simulink model "Scenario_13_CoDeSys"  (R2012b)
settings: Solver=ode3  StartTime=0.0  StopTime=inf  FixedStep=Sample_Time_Model  RelTol=1e-3
PreLoadFcn:
  | Variablen_Scenario13
InitFcn:
  | BT = randperm(9);
values from neighbouring files (symbols this model uses):
  Band_Geschwindigkeit = 1.47    [Variablen_Scenario13.m]
  Band_Sensor_Hell_2_Z = -6.5    [Variablen_Scenario13.m]
  Band_Sensor_Hell_3_Z = -10.36    [Variablen_Scenario13.m]
  Band_Sensor_Hell_4_Z = -14.64    [Variablen_Scenario13.m]
  Band_Sensor_Tolerance_Z = 0.2    [Variablen_Scenario13.m]
  Bauteil_Fallgeschwindigkeit = 0.4    [Variablen_Scenario13.m]
  Bauteil_Farbe_Metall = [0.8 0.8 0.8]    [Variablen_Scenario13.m]
  Bauteil_Farbe_Schwarz = [0.2 0.2 0.2]    [Variablen_Scenario13.m]
  Bauteil_Farbe_Weiss = [1 1 0.2]    [Variablen_Scenario13.m]
  Kran_Dauer_90_Grad = 5    [Variablen_Scenario13.m]
  Kran_Drehwinkel_90_Grad = 8050    [Variablen_Scenario13.m]
  Kran_Sensor_Position_Delta = 0.07    [Variablen_Scenario13.m]
  Sample_Time_Model = 0.05    [Variablen_Scenario13.m]
  Sample_Time_Simulation = 0.1    [Variablen_Scenario13.m]
  Sensor_Band_Metall_1 = -6.5    [Variablen_Scenario13.m]
  Sensor_Band_Metall_2 = -10.36    [Variablen_Scenario13.m]
libraries: simulink x557, vrlib x13, opclib x7, rtwinlib x1
(part 3 of 10)

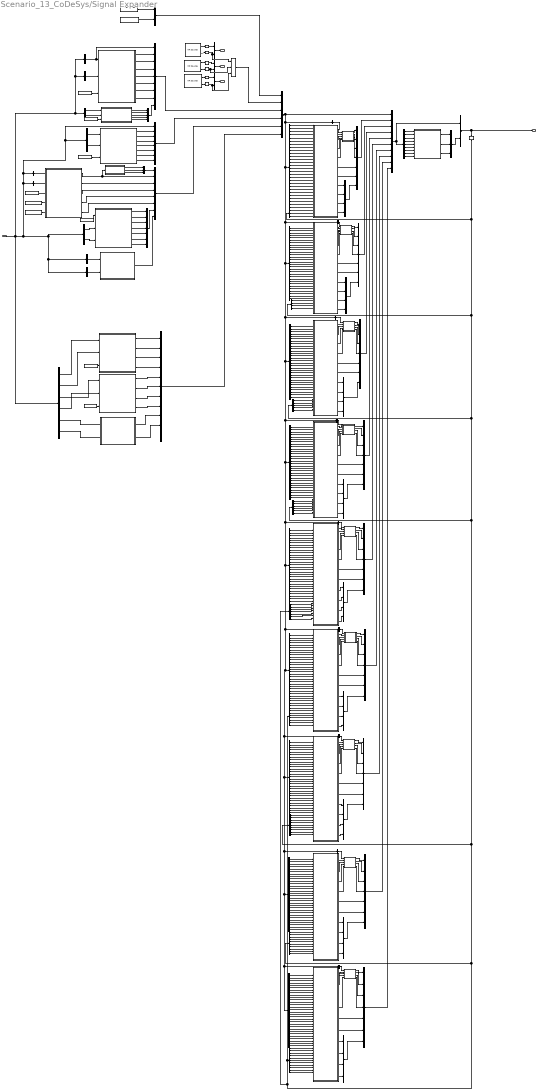
== system Scenario_13_CoDeSys/Signal Expander ==
  In : Inport
  BT_Lager_Status : Subsystem
  Band_Source : vrlib/VR Source  InstantiateOnLoad=on  SampleTime=Sample_Time_Simulation  ViewEnable=on  RemoteChange=off  RemoteView=off  FieldsRead=Switch_5.Button_State.1.1.1.logical#Switch_6.Switch_State.1.1.1.logical  WorldFileName=Visu_Sz_13.wrl  AutoView=off  VideoDimensions=[]  AllowVariableSize=off
  Band_Vor_Zurueck : Stateflow chart  TreatAsAtomicUnit=on
  Band_Zyl_1 : Stateflow chart  TreatAsAtomicUnit=on
  Band_Zyl_2 : Stateflow chart  TreatAsAtomicUnit=on
  Bauteil_1 : Stateflow chart  TreatAsAtomicUnit=on
  Bauteil_2 : Stateflow chart  TreatAsAtomicUnit=on
  Bauteil_3 : Stateflow chart  TreatAsAtomicUnit=on
  Bauteil_4 : Stateflow chart  TreatAsAtomicUnit=on
  Bauteil_5 : Stateflow chart  TreatAsAtomicUnit=on
  Bauteil_6 : Stateflow chart  TreatAsAtomicUnit=on
  Bauteil_7 : Stateflow chart  TreatAsAtomicUnit=on
  Bauteil_8 : Stateflow chart  TreatAsAtomicUnit=on
  Bauteil_9 : Stateflow chart  TreatAsAtomicUnit=on
  Bauteil_Fallgeschwindigkeit : Constant  Value=Bauteil_Fallgeschwindigkeit
  Berechne Band Geschwindigkeit : Subsystem
  Bus Creator : BusCreator  Inputs=5
  Bus Creator1 : BusCreator  Inputs=9
  Bus Creator10 : BusCreator  Inputs=10
  Bus Creator{9,11,21,24,26,29,31,33,35} (9 alike) : BusCreator
  Bus Creator{7..8,12,22,25,27..28,30,32,34} (10 alike) : BusCreator  Inputs=7
  Bus Creator13 : BusCreator  Inputs=3
  Bus Creator{14,18..19,23,36} (5 alike) : BusCreator  Inputs=2
  Bus Creator2 : BusCreator  Inputs=6
  Bus Creator3 : BusCreator  Inputs=8
  Bus Creator4 : BusCreator  Inputs=8
  Bus Creator5 : BusCreator  Inputs=11
  Bus Creator6 : BusCreator  Inputs=3
  Bus Selector1 : BusSelector  OutputSignals=Lager.Lager_X_Achse,Lager.Lager_Ver_Ausgefahren,Kran.Kran_Sensoren.Sensor_Kran_Stellung_Lager,Kran.Kran_Sensoren.Sensor_Kran_Stellung_Band,Kran.Kran_Sensoren.Sensor_Kran_Stellung_Stempel,Kran.Kran_Zyl.Kran_Zyl_Oben,Kran.Kran_Zyl.Kran_Zyl_Unten,Kran.Kran_Sauger,Kran.Kran_Zyl.Kran_Hochheben,Kran.Kran_Zyl.Kran_Runterlassen,Kran.Kran_Drehen_Links_FS,Kran.Kran_Drehen_Rechts_FS,Stempel.Stempel_Halterung_Ausfahren_FS,Stempel.Stempel_Halterung_Einfahren_FS,Band.Band_Vor_FS,Band.Band_Zurueck_FS,Band.Band_Zyl_1_X_Achse,Band.Band_Zyl_2_X_Achse,Lager.Lager_Ver_Ausfahren,Lager.Lager_Vereinzler_Schritt_Aus,Kran.Kran_Zyl.Kran_Zyl_Schritt_Hoch,Kran.Kran_Zyl.Kran_Zyl_Schritt_Runter,Kran.Kran_Drehen_Schritt,Stempel.Stempel_Halterung_Schritt_Aus,Stempel.Stempel_Halterung_Schritt_Ein,Band.Band_Zyl_1_Schritt,Band.Band_Zyl_2_Schritt,Konstante.Band_Geschwindigkeit
  Bus Selector10 : BusSelector  OutputSignals=Stempel.Stempel_Halterung_ausfahren
  Bus Selector11 : BusSelector  OutputSignals=Stempel.Stempel_Halterung_einfahren
  Bus Selector12 : BusSelector  OutputSignals=Stempel.Stempel_einfahren,Stempel.Stempel_ausfahren
  Bus Selector13 : BusSelector  OutputSignals=Kran.Kran_Sauger_An
  Bus Selector14 : BusSelector  OutputSignals=Kran.Kran_Sauger_Aus
  Bus Selector15 : BusSelector  OutputSignals=Kran.Kran_einfahren,Kran.Kran_ausfahren
  Bus Selector16 : BusSelector  OutputSignals=Kran.Kran_Drehen_Links
  Bus Selector17 : BusSelector  OutputSignals=Kran.Kran_Drehen_Rechts
  Bus Selector18 : BusSelector  OutputSignals=Lager.Lager_Zyl_einfahren,Lager.Lager_Zyl_ausfahren
  Bus Selector19 : BusSelector  OutputSignals=Lager.Lager_1_Status,Lager.Lager_2_Status,Lager.Lager_3_Status,Stempelanlage_BT.Bauteil_1.BT_1_Bereit,Stempelanlage_BT.Bauteil_2.BT_2_Bereit
  Bus Selector{2,9,21,23,25,31..32,34} (8 alike) : BusSelector  OutputSignals=Lager.Lager_X_Achse,Lager.Lager_Ver_Eingefahren,Lager.Lager_Ver_Ausgefahren,Kran.Kran_Sensoren.Sensor_Kran_Stellung_Lager,Kran.Kran_Sensoren.Sensor_Kran_Stellung_Band,Kran.Kran_Sensoren.Sensor_Kran_Stellung_Stempel,Kran.Kran_Zyl.Kran_Zyl_Oben,Kran.Kran_Zyl.Kran_Zyl_Unten,Kran.Kran_Sauger,Kran.Kran_Zyl.Kran_Hochheben,Kran.Kran_Zyl.Kran_Runterlassen,Kran.Kran_Drehen_Links_FS,Kran.Kran_Drehen_Rechts_FS,Stempel.Stempel_Halterung_Ausfahren_FS,Stempel.Stempel_Halterung_Einfahren_FS,Band.Band_Vor_FS,Band.Band_Zurueck_FS,Band.Band_Zyl_1_X_Achse,Band.Band_Zyl_2_X_Achse,Lager.Lager_Ver_Ausfahren,Lager.Lager_Vereinzler_Schritt_Aus,Kran.Kran_Zyl.Kran_Zyl_Schritt_Hoch,Kran.Kran_Zyl.Kran_Zyl_Schritt_Runter,Kran.Kran_Drehen_Schritt,Stempel.Stempel_Halterung_Schritt_Aus,Stempel.Stempel_Halterung_Schritt_Ein,Band.Band_Zyl_1_Schritt,Band.Band_Zyl_2_Schritt,Konstante.Band_Geschwindigkeit,Konstante.Bauteil_Fallgeschwindigkeit
  Bus Selector20 : BusSelector  OutputSignals=Lager.Lager_1_Status,Lager.Lager_2_Status,Lager.Lager_3_Status,Stempelanlage_BT.Bauteil_1.BT_1_Bereit,Stempelanlage_BT.Bauteil_2.BT_2_Bereit,Stempelanlage_BT.Bauteil_3.BT_3_Bereit
  Bus Selector22 : BusSelector  OutputSignals=Lager.Lager_1_Status,Lager.Lager_2_Status,Lager.Lager_3_Status,Stempelanlage_BT.Bauteil_1.BT_1_Bereit,Stempelanlage_BT.Bauteil_2.BT_2_Bereit,Stempelanlage_BT.Bauteil_3.BT_3_Bereit,Stempelanlage_BT.Bauteil_4.BT_4_Bereit
  Bus Selector24 : BusSelector  OutputSignals=Lager.Lager_1_Status,Lager.Lager_2_Status,Lager.Lager_3_Status,Stempelanlage_BT.Bauteil_1.BT_1_Bereit,Stempelanlage_BT.Bauteil_2.BT_2_Bereit,Stempelanlage_BT.Bauteil_3.BT_3_Bereit,Stempelanlage_BT.Bauteil_4.BT_4_Bereit,Stempelanlage_BT.Bauteil_5.BT_5_Bereit
  Bus Selector26 : BusSelector  OutputSignals=Band.Band_Zyl_1_einfahren,Band.Band_Zyl_1_ausfahren,Band.Band_Zyl_2_einfahren,Band.Band_Zyl_2_ausfahren,Band.Band_vor,Band.Band_zurueck
  Bus Selector{6,8,27..30,36..38} (9 alike) : BusSelector  OutputSignals=Notaus_Switch
  Bus Selector3 : BusSelector  OutputSignals=Lager.Lager_1_Status,Lager.Lager_2_Status,Lager.Lager_3_Status,Stempelanlage_BT.Bauteil_1.BT_1_Bereit
  Bus Selector33 : BusSelector  OutputSignals=Lager.Lager_1_Status,Lager.Lager_2_Status,Lager.Lager_3_Status,Stempelanlage_BT.Bauteil_1.BT_1_Bereit,Stempelanlage_BT.Bauteil_2.BT_2_Bereit,Stempelanlage_BT.Bauteil_3.BT_3_Bereit,Stempelanlage_BT.Bauteil_4.BT_4_Bereit,Stempelanlage_BT.Bauteil_5.BT_5_Bereit,Stempelanlage_BT.Bauteil_6.BT_6_Bereit,Stempelanlage_BT.Bauteil_7.BT_7_Bereit
  Bus Selector35 : BusSelector  OutputSignals=Lager.Lager_1_Status,Lager.Lager_2_Status,Lager.Lager_3_Status,Stempelanlage_BT.Bauteil_1.BT_1_Bereit,Stempelanlage_BT.Bauteil_2.BT_2_Bereit,Stempelanlage_BT.Bauteil_3.BT_3_Bereit,Stempelanlage_BT.Bauteil_4.BT_4_Bereit,Stempelanlage_BT.Bauteil_5.BT_5_Bereit,Stempelanlage_BT.Bauteil_6.BT_6_Bereit,Stempelanlage_BT.Bauteil_7.BT_7_Bereit,Stempelanlage_BT.Bauteil_8.BT_8_Bereit
  Bus Selector4 : BusSelector  OutputSignals=Bauteil_1.BT_1_Lager,Bauteil_2.BT_2_Lager,Bauteil_3.BT_3_Lager,Bauteil_4.BT_4_Lager,Bauteil_5.BT_5_Lager,Bauteil_6.BT_6_Lager,Bauteil_7.BT_7_Lager,Bauteil_8.BT_8_Lager,Bauteil_9.BT_9_Lager
  Bus Selector5 : BusSelector  OutputSignals=Lager.Lager_1_Status,Lager.Lager_2_Status,Lager.Lager_3_Status
  Bus Selector7 : BusSelector  OutputSignals=Lager.Lager_1_Status,Lager.Lager_2_Status,Lager.Lager_3_Status,Stempelanlage_BT.Bauteil_1.BT_1_Bereit,Stempelanlage_BT.Bauteil_2.BT_2_Bereit,Stempelanlage_BT.Bauteil_3.BT_3_Bereit,Stempelanlage_BT.Bauteil_4.BT_4_Bereit,Stempelanlage_BT.Bauteil_5.BT_5_Bereit,Stempelanlage_BT.Bauteil_6.BT_6_Bereit
  Constant{14..17,24..25,30} (7 alike) : Constant  Value=Sample_Time_Model
  Constant31 : Constant  Value=Kran_Drehwinkel_90_Grad
  Constant32 : Constant  Value=Kran_Dauer_90_Grad
  Halterung_Stempel : Stateflow chart  TreatAsAtomicUnit=on
  Kran : Stateflow chart  TreatAsAtomicUnit=on
  Kran_Position_Sensor : Subsystem
  Kran_Sauger : Stateflow chart  TreatAsAtomicUnit=on
  Kran_Zylinder : Stateflow chart  TreatAsAtomicUnit=on
  Lager : Stateflow chart  TreatAsAtomicUnit=on
  Lager_Source : vrlib/VR Source  InstantiateOnLoad=on  SampleTime=Sample_Time_Simulation  ViewEnable=on  RemoteChange=off  RemoteView=off  FieldsRead=Switch_1.Button_State.1.1.1.logical#Switch_2.Switch_State.1.1.1.logical  WorldFileName=Visu_Sz_13.wrl  AutoView=off  VideoDimensions=[]  AllowVariableSize=off
  Logical Operator : Logic  Operator=OR  Inputs=3  AllPortsSameDT=off  OutDataTypeStr=boolean
  Memory4 : Memory
  Rate Transition{1..6} (6 alike) : RateTransition
  Stempel_Source : vrlib/VR Source  InstantiateOnLoad=on  SampleTime=Sample_Time_Simulation  ViewEnable=on  RemoteChange=off  RemoteView=off  FieldsRead=Switch_3.Button_State.1.1.1.logical#Switch_4.Switch_State.1.1.1.logical  WorldFileName=Visu_Sz_13.wrl  AutoView=off  VideoDimensions=[]  AllowVariableSize=off
  Subsystem : Subsystem
  Subsystem1 : Subsystem
  Subsystem2 : Subsystem
  Subsystem3 : Subsystem
  Subsystem4 : Subsystem
  Subsystem5 : Subsystem
  Subsystem6 : Subsystem
  Subsystem7 : Subsystem
  Subsystem8 : Subsystem
  Zylinder_Stempel : Stateflow chart  TreatAsAtomicUnit=on
  Band_Schalter : Outport
  Lager_Schalter : Outport  Port=2
  Stempel_Schalter : Outport  Port=3
  Bauteil_Ausgang : Outport  Port=4
  wires:
  Halterung_Stempel/1(Halterung_X_Achse) -> Bus Creator1/2  "Stempel_Halterung_X_Achse"
  Bus Creator1/1 -> Bus Creator2/3  "Stempel"
  Lager/1(Vereinzler_X_Achse) -> Bus Creator3/2  "Lager_X_Achse"
  Bus Creator3/1 -> Bus Creator2/4  "Lager"
  Bus Selector18/2 -> Lager/2(Vereinzler_Ausfahren)  "<Lager_Zyl_ausfahren>"
  Bus Selector16/1 -> Kran/1(Kran_Drehen_Links)  "<Kran_Drehen_Links>"
  Bus Creator4/1 -> Bus Creator2/5  "Kran"
  Kran/1(Kran_Stellung) -> Kran_Position_Sensor/1(In), Bus Creator4/2  "Kran_Stellung"
  Bus Selector17/1 -> Kran/2(Kran_Drehen_Rechts)  "<Kran_Drehen_Rechts>"
  Bus Creator5/1 -> Bus Creator2/6  "Band"
  Zylinder_Stempel/1(Zylinder_Y_Achse) -> Bus Creator/1  "Stempel_Zyl_Y"
  Band_Zyl_1/1(Zyl_1_X_Achse) -> Bus Creator5/1  "Band_Zyl_1_X_Achse"
  Band_Zyl_2/2(Zyl_2_X_Achse) -> Bus Creator5/6  "Band_Zyl_2_X_Achse"
  Bus Selector15/1 -> Kran_Zylinder/2(Kran_Zyl_Runter)  "<Kran_einfahren>"
  Kran_Sauger/1(Kran_Sauger_On) -> Bus Creator4/8  "Kran_Sauger"
  Bus Selector13/1 -> Kran_Sauger/1(Kran_Sauger_An)  "<Kran_Sauger_An>"
  Bus Selector14/1 -> Kran_Sauger/2(Kran_Sauger_Aus)  "<Kran_Sauger_Aus>"
  Kran_Position_Sensor/2(Sensor_Kran_Stellung_Band) -> Bus Creator6/2  "Sensor_Kran_Stellung_Band"
  Kran_Position_Sensor/1(Sensor_Kran_Stellung_Lager) -> Bus Creator6/1  "Sensor_Kran_Stellung_Lager"
  Kran_Position_Sensor/3(Sensor_Kran_Stellung_Stempel) -> Bus Creator6/3  "Sensor_Kran_Stellung_Stempel"
  Bus Creator6/1 -> Bus Creator4/1  "Kran_Sensoren"
  Kran_Zylinder/1(Kran_Zyl_Y_Achse) -> Bus Creator7/1  "Kran_Zyl_Y_Achse"
  Kran_Zylinder/2(Kran_Zyl_Oben) -> Bus Creator7/2  "Kran_Zyl_Oben"
  Kran_Zylinder/3(Kran_Zyl_Unten) -> Bus Creator7/3  "Kran_Zyl_Unten"
  Bus Creator7/1 -> Bus Creator4/7  "Kran_Zyl"
  Bus Selector10/1 -> Bus Creator1/1, Halterung_Stempel/1(Halterung_Ausfahren)  "<Stempel_Halterung_ausfahren>"
  Bus Selector11/1 -> Halterung_Stempel/2(Halterung_Einfahren)  "<Stempel_Halterung_einfahren>"
  Bus Selector12/1 -> Zylinder_Stempel/1(Stempel_Einfahren)  "<Stempel_einfahren>"
  Halterung_Stempel/2(Stempel_Halterung_Ausgefahren) -> Bus Creator1/3  "Stempel_Halterung_Ausgefahren"
  Halterung_Stempel/3(Stempel_Halterung_Eingefahren) -> Bus Creator1/4  "Stempel_Halterung_Eingefahren"
  Zylinder_Stempel/2(Stempel_Zylinder_Eingefahren) -> Bus Creator/2  "Stempel_Zyl_Eingefahren"
  Zylinder_Stempel/3(Stempel_Zylinder_Ausgefahren) -> Bus Creator/3  "Stempel_Zyl_Ausgefahren"
  Bus Creator/1 -> Bus Creator1/9  "Stempel_Zyl"
  Bauteil_1/1(BT_Y_Achse) -> Subsystem/2(BT_Y_In)  "BT_1_Y_Achse"
  Bauteil_1/5(BT_X_Achse) -> Bus Creator8/5  "BT_1_X_Achse"
  Bauteil_1/6(BT_Z_Achse) -> Bus Creator8/6  "BT_1_Z_Achse"
  Bus Selector1/1 -> Bauteil_1/1(Lager_X_Achse)  "<Lager_X_Achse>"
  Lager/2(Vereinzler_Eingefahren) -> Bus Creator3/3  "Lager_Ver_Eingefahren"
  Lager/3(Vereinzler_Ausgefahren) -> Bus Creator3/4  "Lager_Ver_Ausgefahren"
  Bus Selector1/2 -> Bauteil_1/2(Lager_Ver_Ausgefahren)  "<Lager_Ver_Ausgefahren>"
  Bus Selector1/3 -> Bauteil_1/3(Kran_Stellung_Lager)  "<Sensor_Kran_Stellung_Lager>"
  Bus Selector1/4 -> Bauteil_1/4(Kran_Stellung_Band)  "<Sensor_Kran_Stellung_Band>"
  Bus Selector1/5 -> Bauteil_1/5(Kran_Stellung_Stempel)  "<Sensor_Kran_Stellung_Stempel>"
  Bus Selector1/6 -> Bauteil_1/6(Kran_Zyl_Oben)  "<Kran_Zyl_Oben>"
  Bus Selector1/7 -> Bauteil_1/7(Kran_Zyl_Unten)  "<Kran_Zyl_Unten>"
  Kran_Zylinder/4(Kran_Hochheben) -> Bus Creator7/4  "Kran_Hochheben"
  Kran_Zylinder/5(Kran_Runterlassen) -> Bus Creator7/5  "Kran_Runterlassen"
  Bus Selector1/9 -> Bauteil_1/9(Kran_Hochheben)  "<Kran_Hochheben>"
  Bus Selector1/10 -> Bauteil_1/10(Kran_Runterlassen)  "<Kran_Runterlassen>"
  Kran/2(Kran_Drehen_Links_FS) -> Bus Creator4/3  "Kran_Drehen_Links_FS"
  Kran/3(Kran_Drehen_Rechts_FS) -> Bus Creator4/4  "Kran_Drehen_Rechts_FS"
  Bus Selector1/11 -> Bauteil_1/11(Kran_Drehen_Links)  "<Kran_Drehen_Links_FS>"
  Bus Selector1/12 -> Bauteil_1/12(Kran_Drehen_Rechts)  "<Kran_Drehen_Rechts_FS>"
  Halterung_Stempel/4(Stempel_Halterung_Ausfahren_FS) -> Bus Creator1/5  "Stempel_Halterung_Ausfahren_FS"
  Halterung_Stempel/5(Stempel_Halterung_Einfahren_FS) -> Bus Creator1/6  "Stempel_Halterung_Einfahren_FS"
  Bus Selector1/13 -> Bauteil_1/13(Stempel_Halterung_Ausfahren)  "<Stempel_Halterung_Ausfahren_FS>"
  Bus Selector1/14 -> Bauteil_1/14(Stempel_Halterung_Einfahren)  "<Stempel_Halterung_Einfahren_FS>"
  Band_Vor_Zurueck/1(Band_Vor_FS) -> Bus Creator5/9  "Band_Vor_FS"
  Band_Vor_Zurueck/2(Band_Zurueck_FS) -> Bus Creator5/10  "Band_Zurueck_FS"
  Bus Selector1/15 -> Bauteil_1/15(Band_Vor)  "<Band_Vor_FS>"
  Bus Selector1/16 -> Bauteil_1/16(Band_Zurueck)  "<Band_Zurueck_FS>"
  Bus Selector1/17 -> Bauteil_1/17(Band_Zyl_1_X_Achse)  "<Band_Zyl_1_X_Achse>"
  Bus Selector1/18 -> Bauteil_1/18(Band_Zyl_2_X_Achse)  "<Band_Zyl_2_X_Achse>"
  Bauteil_1/7(BT_Rotation_1) -> Bus Creator9/1
  Bauteil_1/8(BT_Rotation_2) -> Bus Creator9/2
  Bauteil_1/9(BT_Rotation_3) -> Bus Creator9/3
  Bauteil_1/10(BT_Rotation_4) -> Bus Creator9/4
  Bus Creator9/1 -> Bus Creator8/7  "BT_1_Rotation"
  Lager/5(Lager_Ver_Ausfahren) -> Bus Creator3/6  "Lager_Ver_Ausfahren"
  Lager/4(Lager_Ver_Einfahren) -> Bus Creator3/5  "Lager_Ver_Einfahren"
  Bus Selector1/19 -> Bauteil_1/19(Lager_Ver_Ausfahren)  "<Lager_Ver_Ausfahren>"
  Bus Creator8/1 -> Bus Creator10/2  "Bauteil_1"
  Bus Creator10/1 -> Bus Creator14/1, Bus Selector4/1  "Stempelanlage_BT"
  Bauteil_2/7(BT_Rotation_1) -> Bus Creator11/1
  Bauteil_2/8(BT_Rotation_2) -> Bus Creator11/2
  Bauteil_2/9(BT_Rotation_3) -> Bus Creator11/3
  Bauteil_2/10(BT_Rotation_4) -> Bus Creator11/4
  Bauteil_2/5(BT_X_Achse) -> Bus Creator12/5  "BT_2_X_Achse"
  Bauteil_2/1(BT_Y_Achse) -> Subsystem8/2(BT_Y_In)  "BT_2_Y_Achse"
  Bauteil_2/6(BT_Z_Achse) -> Bus Creator12/6  "BT_2_Z_Achse"
  Bus Creator11/1 -> Bus Creator12/7  "BT_2_Rotation"
  Bus Creator12/1 -> Bus Creator10/3  "Bauteil_2"
  Bauteil_1/4(BT_1_Bereit) -> Subsystem/5(BT_Bereit)
  Bauteil_1/2(BT_1_Lager) -> Subsystem/3(BT_Lager_In)  "BT_1_Lager"
  Bauteil_2/2(BT_Lager) -> Subsystem8/3(BT_Lager_In)
  Bus Selector4/1 -> BT_Lager_Status/1(BT_1_Lager_Position)  "<BT_1_Lager>"
  Bus Selector4/2 -> BT_Lager_Status/2(BT_2_Lager_Position)  "<BT_2_Lager>"
  BT_Lager_Status/1(Lager_1_Status) -> Bus Creator13/1  "Lager_1_Status"
  BT_Lager_Status/2(Lager_2_Status) -> Bus Creator13/2  "Lager_2_Status"
  BT_Lager_Status/3(Lager_3_Status) -> Bus Creator13/3  "Lager_3_Status"
  Bus Creator14/1 -> Bauteil_Ausgang/1, Memory4/1
  Bus Creator13/1 -> Bus Creator14/2  "Lager"
  Bauteil_2/4(BT_Bereit) -> Subsystem8/5(BT_Bereit)
  Bus Selector5/1 -> Bauteil_1/29(Lager_1_Status)  "<Lager_1_Status>"
  Bus Selector5/2 -> Bauteil_1/30(Lager_2_Status)  "<Lager_2_Status>"
  Bus Selector5/3 -> Bauteil_1/31(Lager_3_Status)  "<Lager_3_Status>"
  In/1 -> Bus Selector26/1, Bus Selector10/1, Bus Selector11/1, Bus Selector12/1, Bus Creator3/1, Bus Selector18/1, Bus Selector16/1, Bus Selector17/1, Bus Selector13/1, Bus Selector14/1, Bus Selector15/1  "Kran_Lager_FS"
  Band_Zyl_2/4(Band_Zyl_2_Ausgefahren) -> Bus Creator5/8  "Band_Zyl_2_Ausgefahren"
  Band_Zyl_2/3(Band_Zyl_2_Eingefahren) -> Bus Creator5/7  "Band_Zyl_2_Eingefahren"
  Band_Zyl_1/2(Band_Zyl_1_Eingefahren) -> Bus Creator5/2  "Band_Zyl_1_Eingefahren"
  Band_Zyl_1/3(Band_Zyl_1_Ausgefahren) -> Bus Creator5/3  "Band_Zyl_1_Ausgefahren"
  Bauteil_1/3(Kran_Sauger_BT) -> Subsystem/4(BT_angesaugt_in)  "Kran_Sauger_BT_1"
  Bauteil_2/3(Kran_Sauger_BT) -> Subsystem8/4(BT_angesaugt_in)
  Bus Creator21/1 -> Bus Creator22/7  "BT_3_Rotation"
  Bauteil_3/5(BT_X_Achse) -> Bus Creator22/5  "BT_3_X_Achse"
  Bauteil_3/1(BT_Y_Achse) -> Subsystem1/2(BT_Y_In)
  Bauteil_3/6(BT_Z_Achse) -> Bus Creator22/6  "BT_3_Z_Achse"
  Bauteil_3/4(BT_Bereit) -> Subsystem1/5(BT_Bereit)
  Bauteil_3/2(BT_Lager) -> Subsystem1/3(BT_Lager_In)
  Bauteil_3/3(Kran_Sauger_BT) -> Subsystem1/4(BT_angesaugt_in)
  Bauteil_3/7(BT_Rotation_1) -> Bus Creator21/1
  Bauteil_3/8(BT_Rotation_2) -> Bus Creator21/2
  Bauteil_3/9(BT_Rotation_3) -> Bus Creator21/3
  Bauteil_3/10(BT_Rotation_4) -> Bus Creator21/4
  Bus Creator22/1 -> Bus Creator10/4  "Bauteil_3"
  Bus Selector4/3 -> BT_Lager_Status/3(BT_3_Lager_Position)  "<BT_3_Lager>"
  Constant14/1 -> Lager/3(Sample_Time)
  Constant15/1 -> Halterung_Stempel/3(Sample_Time)
  Constant16/1 -> Zylinder_Stempel/3(Sample_Time)
  Constant17/1 -> Kran_Zylinder/1(Sample_Time)
  Constant24/1 -> Kran/3(Sample_Time)
  Constant25/1 -> Band_Zyl_1/3(Sample_Time)
  Constant30/1 -> Band_Zyl_2/3(Sample_Time)
  Halterung_Stempel/6(Schrittgroesse_Ausfahren) -> Bus Creator1/7  "Stempel_Halterung_Schritt_Aus"
  Halterung_Stempel/7(Schrittgroesse_Einfahren) -> Bus Creator1/8  "Stempel_Halterung_Schritt_Ein"
  Zylinder_Stempel/4(Schrittgroesse_Ausfahren) -> Bus Creator/4  "Stempel_Zyl_Schritt_Aus"
  Zylinder_Stempel/5(Schrittgroesse_Einfahren) -> Bus Creator/5  "Stempel_Zyl_Schritt_Ein"
  Lager/6(Schrittgroesse_Ausfahren) -> Bus Creator3/7  "Lager_Vereinzler_Schritt_Aus"
  Lager/7(Schrittgroesse_Einfahren) -> Bus Creator3/8  "Lager_Vereinzler_Schritt_Ein"
  Kran/4(Schrittgroesse_Drehen) -> Bus Creator4/5  "Kran_Drehen_Schritt"
  Kran_Zylinder/6(Schrittgroesse_Ausfahren) -> Bus Creator7/6  "Kran_Zyl_Schritt_Runter"
  Kran_Zylinder/7(Schrittgroesse_Einfahren) -> Bus Creator7/7  "Kran_Zyl_Schritt_Hoch"
  Band_Zyl_2/1(Schrittgroesse) -> Bus Creator5/5  "Band_Zyl_2_Schritt"
  Band_Zyl_1/4(Schrittgroesse) -> Bus Creator5/4  "Band_Zyl_1_Schritt"
  Bus Selector1/20 -> Bauteil_1/20(Lager_Vereinzler_Schritt_Aus)  "<Lager_Vereinzler_Schritt_Aus>"
  Bus Selector1/22 -> Bauteil_1/22(Kran_Zyl_Schritt_Runter)  "<Kran_Zyl_Schritt_Runter>"
  Bus Selector1/21 -> Bauteil_1/21(Kran_Zyl_Schritt_Hoch)  "<Kran_Zyl_Schritt_Hoch>"
  Bus Selector1/23 -> Bauteil_1/23(Kran_Drehen_Schritt)  "<Kran_Drehen_Schritt>"
  Bus Selector1/24 -> Bauteil_1/24(Stempel_Halterung_Schritt_Aus)  "<Stempel_Halterung_Schritt_Aus>"
  Bus Selector1/25 -> Bauteil_1/25(Stempel_Halterung_Schritt_Ein)  "<Stempel_Halterung_Schritt_Ein>"
  Bus Selector1/8 -> Bauteil_1/8(Kran_Sauger)  "<Kran_Sauger>"
  Bus Selector1/26 -> Bauteil_1/26(Band_Zyl_1_Schritt)  "<Band_Zyl_1_Schritt>"
  Bus Selector1/27 -> Bauteil_1/27(Band_Zyl_2_Schritt)  "<Band_Zyl_2_Schritt>"
  Berechne Band Geschwindigkeit/1(Band_Geschwindigkeit) -> Bus Creator23/1  "Band_Geschwindigkeit"
  Bauteil_Fallgeschwindigkeit/1 -> Bus Creator23/2  "Bauteil_Fallgeschwindigkeit"
  Bus Creator23/1 -> Bus Creator2/1  "Konstante"
  Bus Selector1/28 -> Bauteil_1/28(Band_Geschwindigkeit)  "<Band_Geschwindigkeit>"
  Bus Selector2/10 -> Bauteil_2/10(Kran_Hochheben)  "<Kran_Hochheben>"
  Bus Selector2/28 -> Bauteil_2/28(Band_Zyl_2_Schritt)  "<Band_Zyl_2_Schritt>"
  Bus Selector2/11 -> Bauteil_2/11(Kran_Runterlassen)  "<Kran_Runterlassen>"
  Bus Selector2/7 -> Bauteil_2/7(Kran_Zyl_Oben)  "<Kran_Zyl_Oben>"
  Bus Selector2/3 -> Bauteil_2/3(Lager_Ver_Ausgefahren)  "<Lager_Ver_Ausgefahren>"
  Bus Selector3/2 -> Bauteil_2/32(Lager_2_Status)  "<Lager_2_Status>"
  Bus Selector3/1 -> Bauteil_2/31(Lager_1_Status)  "<Lager_1_Status>"
  Bus Selector2/4 -> Bauteil_2/4(Kran_Stellung_Lager)  "<Sensor_Kran_Stellung_Lager>"
  Bus Selector2/30 -> Bauteil_2/30(Bauteil_Fallgeschwindigkeit)  "<Bauteil_Fallgeschwindigkeit>"
  Bus Selector2/21 -> Bauteil_2/21(Lager_Vereinzler_Schritt_Aus)  "<Lager_Vereinzler_Schritt_Aus>"
  Bus Selector2/8 -> Bauteil_2/8(Kran_Zyl_Unten)  "<Kran_Zyl_Unten>"
  Bus Selector2/23 -> Bauteil_2/23(Kran_Zyl_Schritt_Runter)  "<Kran_Zyl_Schritt_Runter>"
  Bus Selector2/6 -> Bauteil_2/6(Kran_Stellung_Stempel)  "<Sensor_Kran_Stellung_Stempel>"
  Bus Selector2/1 -> Bauteil_2/1(Lager_X_Achse)  "<Lager_X_Achse>"
  Bus Selector2/27 -> Bauteil_2/27(Band_Zyl_1_Schritt)  "<Band_Zyl_1_Schritt>"
  Bus Selector2/13 -> Bauteil_2/13(Kran_Drehen_Rechts)  "<Kran_Drehen_Rechts_FS>"
  Bus Selector2/15 -> Bauteil_2/15(Stempel_Halterung_Einfahren)  "<Stempel_Halterung_Einfahren_FS>"
  Bus Selector2/19 -> Bauteil_2/19(Band_Zyl_2_X_Achse)  "<Band_Zyl_2_X_Achse>"
  Bus Selector2/18 -> Bauteil_2/18(Band_Zyl_1_X_Achse)  "<Band_Zyl_1_X_Achse>"
  Bus Selector2/22 -> Bauteil_2/22(Kran_Zyl_Schritt_Hoch)  "<Kran_Zyl_Schritt_Hoch>"
  Bus Selector2/20 -> Bauteil_2/20(Lager_Ver_Ausfahren)  "<Lager_Ver_Ausfahren>"
  Bus Selector2/17 -> Bauteil_2/17(Band_Zurueck)  "<Band_Zurueck_FS>"
  Bus Selector2/24 -> Bauteil_2/24(Kran_Drehen_Schritt)  "<Kran_Drehen_Schritt>"
  Bus Selector2/14 -> Bauteil_2/14(Stempel_Halterung_Ausfahren)  "<Stempel_Halterung_Ausfahren_FS>"
  Bus Selector2/16 -> Bauteil_2/16(Band_Vor)  "<Band_Vor_FS>"
  Bus Selector2/25 -> Bauteil_2/25(Stempel_Halterung_Schritt_Aus)  "<Stempel_Halterung_Schritt_Aus>"
  Bus Selector2/2 -> Bauteil_2/2(Lager_Ver_Eingefahren)  "<Lager_Ver_Eingefahren>"
  Bus Selector2/26 -> Bauteil_2/26(Stempel_Halterung_Schritt_Ein)  "<Stempel_Halterung_Schritt_Ein>"
  Bus Selector2/9 -> Bauteil_2/9(Kran_Sauger)  "<Kran_Sauger>"
  Bus Selector2/29 -> Bauteil_2/29(Band_Geschwindigkeit)  "<Band_Geschwindigkeit>"
  Bus Selector3/3 -> Bauteil_2/33(Lager_3_Status)  "<Lager_3_Status>"
  Bus Selector2/12 -> Bauteil_2/12(Kran_Drehen_Links)  "<Kran_Drehen_Links_FS>"
  Bus Selector2/5 -> Bauteil_2/5(Kran_Stellung_Band)  "<Sensor_Kran_Stellung_Band>"
  Bus Selector3/4 -> Bauteil_2/34(BT_1_Bereit)  "<BT_1_Bereit>"
  Bus Selector19/4 -> Bauteil_3/34(BT_1_Bereit)  "<BT_1_Bereit>"
  Bus Selector19/2 -> Bauteil_3/32(Lager_2_Status)  "<Lager_2_Status>"
  Bus Selector19/3 -> Bauteil_3/33(Lager_3_Status)  "<Lager_3_Status>"
  Bus Selector19/1 -> Bauteil_3/31(Lager_1_Status)  "<Lager_1_Status>"
  Bus Selector19/5 -> Bauteil_3/35(BT_2_Bereit)  "<BT_2_Bereit>"
  Bus Selector20/4 -> Bauteil_4/34(BT_1_Bereit)  "<BT_1_Bereit>"
  Bus Selector20/5 -> Bauteil_4/35(BT_2_Bereit)  "<BT_2_Bereit>"
  Bus Selector20/2 -> Bauteil_4/32(Lager_2_Status)  "<Lager_2_Status>"
  Bus Selector20/1 -> Bauteil_4/31(Lager_1_Status)  "<Lager_1_Status>"
  Bus Selector20/3 -> Bauteil_4/33(Lager_3_Status)  "<Lager_3_Status>"
  Bauteil_4/6(BT_Z_Achse) -> Bus Creator25/6  "BT_4_Z_Achse"
  Bauteil_4/4(BT_Bereit) -> Subsystem2/5(BT_Bereit)
  Bauteil_4/2(BT_Lager) -> Subsystem2/3(BT_Lager_In)
  Bauteil_4/1(BT_Y_Achse) -> Subsystem2/2(BT_Y_In)  "BT_4_Y_Achse"
  Bauteil_4/3(Kran_Sauger_BT) -> Subsystem2/4(BT_angesaugt_in)
  Bauteil_4/5(BT_X_Achse) -> Bus Creator25/5  "BT_4_X_Achse"
  Bauteil_4/9(BT_Rotation_3) -> Bus Creator24/3
  Bauteil_4/10(BT_Rotation_4) -> Bus Creator24/4
  Bauteil_4/8(BT_Rotation_2) -> Bus Creator24/2
  Bauteil_4/7(BT_Rotation_1) -> Bus Creator24/1
  Bus Creator24/1 -> Bus Creator25/7  "BT_4_Rotation"
  Bus Creator25/1 -> Bus Creator10/5  "Bauteil_4"
  Bus Selector20/6 -> Bauteil_4/36(BT_3_Bereit)  "<BT_3_Bereit>"
  Bus Selector22/6 -> Bauteil_5/36(BT_3_Bereit)  "<BT_3_Bereit>"
  Bus Selector22/5 -> Bauteil_5/35(BT_2_Bereit)  "<BT_2_Bereit>"
  Bus Selector22/1 -> Bauteil_5/31(Lager_1_Status)  "<Lager_1_Status>"
  Bus Selector22/4 -> Bauteil_5/34(BT_1_Bereit)  "<BT_1_Bereit>"
  Bus Selector22/3 -> Bauteil_5/33(Lager_3_Status)  "<Lager_3_Status>"
  Bus Selector22/2 -> Bauteil_5/32(Lager_2_Status)  "<Lager_2_Status>"
  Bauteil_5/6(BT_Z_Achse) -> Bus Creator27/6  "BT_5_Z_Achse"
  Bauteil_5/4(BT_Bereit) -> Subsystem3/5(BT_Bereit)
  Bauteil_5/2(BT_Lager) -> Subsystem3/3(BT_Lager_In)
  Bauteil_5/1(BT_Y_Achse) -> Subsystem3/2(BT_Y_In)  "BT_5_Y_Achse"
  Bauteil_5/3(Kran_Sauger_BT) -> Subsystem3/4(BT_angesaugt_in)
  Bauteil_5/5(BT_X_Achse) -> Bus Creator27/5  "BT_5_X_Achse"
  Bauteil_5/9(BT_Rotation_3) -> Bus Creator26/3
  Bauteil_5/8(BT_Rotation_2) -> Bus Creator26/2
  Bauteil_5/7(BT_Rotation_1) -> Bus Creator26/1
  Bus Creator26/1 -> Bus Creator27/7  "BT_5_Rotation"
  Bauteil_5/10(BT_Rotation_4) -> Bus Creator26/4
  Bus Creator27/1 -> Bus Creator10/6  "Bauteil_5"
  Bus Selector22/7 -> Bauteil_5/37(BT_4_Bereit)  "<BT_4_Bereit>"
  Bus Selector24/4 -> Bauteil_6/34(BT_1_Bereit)  "<BT_1_Bereit>"
  Bus Selector24/1 -> Bauteil_6/31(Lager_1_Status)  "<Lager_1_Status>"
  Bus Selector24/3 -> Bauteil_6/33(Lager_3_Status)  "<Lager_3_Status>"
  Bus Selector24/6 -> Bauteil_6/36(BT_3_Bereit)  "<BT_3_Bereit>"
  Bus Selector24/2 -> Bauteil_6/32(Lager_2_Status)  "<Lager_2_Status>"
  Bus Selector24/5 -> Bauteil_6/35(BT_2_Bereit)  "<BT_2_Bereit>"
  Bauteil_6/7(BT_Rotation_1) -> Bus Creator29/1
  Bauteil_6/8(BT_Rotation_2) -> Bus Creator29/2
  Bauteil_6/9(BT_Rotation_3) -> Bus Creator29/3
  Bauteil_6/10(BT_Rotation_4) -> Bus Creator29/4
  Bauteil_6/5(BT_X_Achse) -> Bus Creator28/5  "BT_6_X_Achse"
  Bauteil_6/1(BT_Y_Achse) -> Subsystem4/2(BT_Y_In)  "BT_6_Y_Achse"
  Bauteil_6/6(BT_Z_Achse) -> Bus Creator28/6  "BT_6_Z_Achse"
  Bauteil_6/4(BT_Bereit) -> Subsystem4/5(BT_Bereit)
  Bauteil_6/2(BT_Lager) -> Subsystem4/3(BT_Lager_In)
  Bauteil_6/3(Kran_Sauger_BT) -> Subsystem4/4(BT_angesaugt_in)
  Bus Creator29/1 -> Bus Creator28/7  "BT_6_Rotation"
  Bus Creator28/1 -> Bus Creator10/7  "Bauteil_6"
  Bus Selector24/8 -> Bauteil_6/38(BT_5_Bereit)  "<BT_5_Bereit>"
  Bus Selector24/7 -> Bauteil_6/37(BT_4_Bereit)  "<BT_4_Bereit>"
  Constant31/1 -> Kran/4(Kran_Drehwinkel_90_Grad)
  Kran/5(Kran_Drehwinkel) -> Bus Creator4/6  "Kran_Drehwinkel"
  Constant32/1 -> Kran/5(Kran_Dauer_90_Grad)
  Bus Selector18/1 -> Lager/1(Vereinzler_Einfahren)  "<Lager_Zyl_einfahren>"
  Bus Selector12/2 -> Zylinder_Stempel/2(Stempel_Ausfahren)  "<Stempel_ausfahren>"
  Bus Selector15/2 -> Kran_Zylinder/3(Kran_Zyl_Hoch)  "<Kran_ausfahren>"
  Bus Selector4/6 -> BT_Lager_Status/6(BT_6_Lager_Position)  "<BT_6_Lager>"
  Bus Selector4/5 -> BT_Lager_Status/5(BT_5_Lager_Position)  "<BT_5_Lager>"
  Bus Selector4/4 -> BT_Lager_Status/4(BT_4_Lager_Position)  "<BT_4_Lager>"
  Rate Transition1/1 -> Bus Creator19/1  "Lager_Start"
  Rate Transition4/1 -> Logical Operator/1, Bus Creator18/2  "Stempel_NotAus"
  Rate Transition3/1 -> Bus Creator18/1  "Stempel_Start"
  Rate Transition5/1 -> Bus Creator36/1  "Band_Start"
  Rate Transition6/1 -> Logical Operator/3, Bus Creator36/2  "Band_NotAus"
  Bus Selector7/4 -> Bauteil_7/34(BT_1_Bereit)  "<BT_1_Bereit>"
  Bus Selector7/1 -> Bauteil_7/31(Lager_1_Status)  "<Lager_1_Status>"
  Bus Selector7/3 -> Bauteil_7/33(Lager_3_Status)  "<Lager_3_Status>"
  Bus Selector7/6 -> Bauteil_7/36(BT_3_Bereit)  "<BT_3_Bereit>"
  Bus Selector7/2 -> Bauteil_7/32(Lager_2_Status)  "<Lager_2_Status>"
  Bus Selector7/5 -> Bauteil_7/35(BT_2_Bereit)  "<BT_2_Bereit>"
  Bus Selector7/8 -> Bauteil_7/38(BT_5_Bereit)  "<BT_5_Bereit>"
  Bus Selector7/7 -> Bauteil_7/37(BT_4_Bereit)  "<BT_4_Bereit>"
  Bus Selector7/9 -> Bauteil_7/39(BT_6_Bereit)  "<BT_6_Bereit>"
  Bauteil_7/7(BT_Rotation_1) -> Bus Creator31/1
  Bauteil_7/8(BT_Rotation_2) -> Bus Creator31/2
  Bauteil_7/9(BT_Rotation_3) -> Bus Creator31/3
  Bauteil_7/10(BT_Rotation_4) -> Bus Creator31/4
  Bauteil_7/5(BT_X_Achse) -> Bus Creator30/5  "BT_7_X_Achse"
  Bauteil_7/1(BT_Y_Achse) -> Subsystem5/2(BT_Y_In)  "BT_7_Y_Achse"
  Bauteil_7/6(BT_Z_Achse) -> Bus Creator30/6  "BT_7_Z_Achse"
  Bauteil_7/4(BT_Bereit) -> Subsystem5/5(BT_Bereit)
  Bauteil_7/2(BT_Lager) -> Subsystem5/3(BT_Lager_In)
  Bauteil_7/3(Kran_Sauger_BT) -> Subsystem5/4(BT_angesaugt_in)
  Bus Creator31/1 -> Bus Creator30/7  "BT_7_Rotation"
  Bus Creator30/1 -> Bus Creator10/8  "Bauteil_7"
  Bus Selector33/4 -> Bauteil_8/34(BT_1_Bereit)  "<BT_1_Bereit>"
  Bus Selector33/1 -> Bauteil_8/31(Lager_1_Status)  "<Lager_1_Status>"
  Bus Selector33/3 -> Bauteil_8/33(Lager_3_Status)  "<Lager_3_Status>"
  Bus Selector33/6 -> Bauteil_8/36(BT_3_Bereit)  "<BT_3_Bereit>"
  Bus Selector33/2 -> Bauteil_8/32(Lager_2_Status)  "<Lager_2_Status>"
  Bus Selector33/5 -> Bauteil_8/35(BT_2_Bereit)  "<BT_2_Bereit>"
  Bus Selector33/8 -> Bauteil_8/38(BT_5_Bereit)  "<BT_5_Bereit>"
  Bus Selector33/7 -> Bauteil_8/37(BT_4_Bereit)  "<BT_4_Bereit>"
  Bus Selector33/9 -> Bauteil_8/39(BT_6_Bereit)  "<BT_6_Bereit>"
  Bauteil_8/7(BT_Rotation_1) -> Bus Creator33/1
  Bauteil_8/8(BT_Rotation_2) -> Bus Creator33/2
  Bauteil_8/9(BT_Rotation_3) -> Bus Creator33/3
  Bauteil_8/10(BT_Rotation_4) -> Bus Creator33/4
  Bauteil_8/5(BT_X_Achse) -> Bus Creator32/5  "BT_8_X_Achse"
  Bauteil_8/1(BT_Y_Achse) -> Subsystem6/2(BT_Y_In)  "BT_8_Y_Achse"
  Bauteil_8/6(BT_Z_Achse) -> Bus Creator32/6  "BT_8_Z_Achse"
  Bauteil_8/4(BT_Bereit) -> Subsystem6/5(BT_Bereit)
  Bauteil_8/2(BT_Lager) -> Subsystem6/3(BT_Lager_In)
  Bauteil_8/3(Kran_Sauger_BT) -> Subsystem6/4(BT_angesaugt_in)
  Bus Creator33/1 -> Bus Creator32/7  "BT_8_Rotation"
  Bus Creator32/1 -> Bus Creator10/9  "Bauteil_8"
  Bus Selector33/10 -> Bauteil_8/40(BT_7_Bereit)  "<BT_7_Bereit>"
  Memory4/1 -> Bus Selector20/1, Bus Selector35/1, Bus Selector24/1, Bus Selector22/1, Bus Selector33/1, Bus Selector7/1, Bus Selector19/1, Bus Selector3/1, Bus Selector5/1
  Bus Selector35/4 -> Bauteil_9/34(BT_1_Bereit)  "<BT_1_Bereit>"
  Bus Selector35/1 -> Bauteil_9/31(Lager_1_Status)  "<Lager_1_Status>"
  Bus Selector35/3 -> Bauteil_9/33(Lager_3_Status)  "<Lager_3_Status>"
  Bus Selector35/6 -> Bauteil_9/36(BT_3_Bereit)  "<BT_3_Bereit>"
  Bus Selector35/2 -> Bauteil_9/32(Lager_2_Status)  "<Lager_2_Status>"
  Bus Selector35/5 -> Bauteil_9/35(BT_2_Bereit)  "<BT_2_Bereit>"
  Bus Selector35/8 -> Bauteil_9/38(BT_5_Bereit)  "<BT_5_Bereit>"
  Bus Selector35/7 -> Bauteil_9/37(BT_4_Bereit)  "<BT_4_Bereit>"
  Bus Selector35/9 -> Bauteil_9/39(BT_6_Bereit)  "<BT_6_Bereit>"
  Bauteil_9/7(BT_Rotation_1) -> Bus Creator35/1
  Bauteil_9/8(BT_Rotation_2) -> Bus Creator35/2
  Bauteil_9/9(BT_Rotation_3) -> Bus Creator35/3
  Bauteil_9/10(BT_Rotation_4) -> Bus Creator35/4
  Bauteil_9/5(BT_X_Achse) -> Bus Creator34/5  "BT_9_X_Achse"
  Bauteil_9/1(BT_Y_Achse) -> Subsystem7/2(BT_Y_In)  "BT_9_Y_Achse"
  Bauteil_9/6(BT_Z_Achse) -> Bus Creator34/6  "BT_9_Z_Achse"
  Bauteil_9/4(BT_Bereit) -> Subsystem7/5(BT_Bereit)
  Bauteil_9/2(BT_Lager) -> Subsystem7/3(BT_Lager_In)
  Bauteil_9/3(Kran_Sauger_BT) -> Subsystem7/4(BT_angesaugt_in)
  Bus Creator35/1 -> Bus Creator34/7  "BT_9_Rotation"
  Bus Creator34/1 -> Bus Creator10/10  "Bauteil_9"
  Bus Selector35/10 -> Bauteil_9/40(BT_7_Bereit)  "<BT_7_Bereit>"
  Bus Selector35/11 -> Bauteil_9/41(BT_8_Bereit)  "<BT_8_Bereit>"
  Bus Selector4/7 -> BT_Lager_Status/7(BT_7_Lager_Position)  "<BT_7_Lager>"
  Bus Selector4/9 -> BT_Lager_Status/9(BT_9_Lager_Position)  "<BT_9_Lager>"
  Bus Selector4/8 -> BT_Lager_Status/8(BT_8_Lager_Position)  "<BT_8_Lager>"
  Bus Selector26/1 -> Band_Zyl_1/1(Zyl_1_Einfahren)  "<Band_Zyl_1_einfahren>"
  Bus Selector26/2 -> Band_Zyl_1/2(Zyl_1_Ausfahren)  "<Band_Zyl_1_ausfahren>"
  Bus Selector26/3 -> Band_Zyl_2/1(Zyl_2_Einfahren)  "<Band_Zyl_2_einfahren>"
  Bus Selector26/4 -> Band_Zyl_2/2(Zyl_2_Ausfahren)  "<Band_Zyl_2_ausfahren>"
  Bus Selector26/5 -> Band_Vor_Zurueck/1(Band_Vor)  "<Band_vor>"
  Bus Selector26/6 -> Band_Vor_Zurueck/2(Band_Zurueck)  "<Band_zurueck>"
  Bus Selector9/10 -> Bauteil_3/10(Kran_Hochheben)  "<Kran_Hochheben>"
  Bus Selector9/28 -> Bauteil_3/28(Band_Zyl_2_Schritt)  "<Band_Zyl_2_Schritt>"
  Bus Selector9/11 -> Bauteil_3/11(Kran_Runterlassen)  "<Kran_Runterlassen>"
  Bus Selector9/7 -> Bauteil_3/7(Kran_Zyl_Oben)  "<Kran_Zyl_Oben>"
  Bus Selector9/3 -> Bauteil_3/3(Lager_Ver_Ausgefahren)  "<Lager_Ver_Ausgefahren>"
  Bus Selector9/4 -> Bauteil_3/4(Kran_Stellung_Lager)  "<Sensor_Kran_Stellung_Lager>"
  Bus Selector9/30 -> Bauteil_3/30(Bauteil_Fallgeschwindigkeit)  "<Bauteil_Fallgeschwindigkeit>"
  Bus Selector9/21 -> Bauteil_3/21(Lager_Vereinzler_Schritt_Aus)  "<Lager_Vereinzler_Schritt_Aus>"
  Bus Selector9/8 -> Bauteil_3/8(Kran_Zyl_Unten)  "<Kran_Zyl_Unten>"
  Bus Selector9/23 -> Bauteil_3/23(Kran_Zyl_Schritt_Runter)  "<Kran_Zyl_Schritt_Runter>"
  Bus Selector9/6 -> Bauteil_3/6(Kran_Stellung_Stempel)  "<Sensor_Kran_Stellung_Stempel>"
  Bus Selector9/1 -> Bauteil_3/1(Lager_X_Achse)  "<Lager_X_Achse>"
  Bus Selector9/27 -> Bauteil_3/27(Band_Zyl_1_Schritt)  "<Band_Zyl_1_Schritt>"
  Bus Selector9/13 -> Bauteil_3/13(Kran_Drehen_Rechts)  "<Kran_Drehen_Rechts_FS>"
  Bus Selector9/15 -> Bauteil_3/15(Stempel_Halterung_Einfahren)  "<Stempel_Halterung_Einfahren_FS>"
  Bus Selector9/19 -> Bauteil_3/19(Band_Zyl_2_X_Achse)  "<Band_Zyl_2_X_Achse>"
  Bus Selector9/18 -> Bauteil_3/18(Band_Zyl_1_X_Achse)  "<Band_Zyl_1_X_Achse>"
  Bus Selector9/22 -> Bauteil_3/22(Kran_Zyl_Schritt_Hoch)  "<Kran_Zyl_Schritt_Hoch>"
  Bus Selector9/20 -> Bauteil_3/20(Lager_Ver_Ausfahren)  "<Lager_Ver_Ausfahren>"
  Bus Selector9/17 -> Bauteil_3/17(Band_Zurueck)  "<Band_Zurueck_FS>"
  Bus Selector9/24 -> Bauteil_3/24(Kran_Drehen_Schritt)  "<Kran_Drehen_Schritt>"
  Bus Selector9/14 -> Bauteil_3/14(Stempel_Halterung_Ausfahren)  "<Stempel_Halterung_Ausfahren_FS>"
  Bus Selector9/16 -> Bauteil_3/16(Band_Vor)  "<Band_Vor_FS>"
  Bus Selector9/25 -> Bauteil_3/25(Stempel_Halterung_Schritt_Aus)  "<Stempel_Halterung_Schritt_Aus>"
  Bus Selector9/2 -> Bauteil_3/2(Lager_Ver_Eingefahren)  "<Lager_Ver_Eingefahren>"
  Bus Selector9/26 -> Bauteil_3/26(Stempel_Halterung_Schritt_Ein)  "<Stempel_Halterung_Schritt_Ein>"
  Bus Selector9/9 -> Bauteil_3/9(Kran_Sauger)  "<Kran_Sauger>"
  Bus Selector9/29 -> Bauteil_3/29(Band_Geschwindigkeit)  "<Band_Geschwindigkeit>"
  Bus Selector9/12 -> Bauteil_3/12(Kran_Drehen_Links)  "<Kran_Drehen_Links_FS>"
  Bus Selector9/5 -> Bauteil_3/5(Kran_Stellung_Band)  "<Sensor_Kran_Stellung_Band>"
  Bus Selector21/10 -> Bauteil_4/10(Kran_Hochheben)  "<Kran_Hochheben>"
  Bus Selector21/28 -> Bauteil_4/28(Band_Zyl_2_Schritt)  "<Band_Zyl_2_Schritt>"
  Bus Selector21/11 -> Bauteil_4/11(Kran_Runterlassen)  "<Kran_Runterlassen>"
  Bus Selector21/7 -> Bauteil_4/7(Kran_Zyl_Oben)  "<Kran_Zyl_Oben>"
  Bus Selector21/3 -> Bauteil_4/3(Lager_Ver_Ausgefahren)  "<Lager_Ver_Ausgefahren>"
  Bus Selector21/4 -> Bauteil_4/4(Kran_Stellung_Lager)  "<Sensor_Kran_Stellung_Lager>"
  Bus Selector21/30 -> Bauteil_4/30(Bauteil_Fallgeschwindigkeit)  "<Bauteil_Fallgeschwindigkeit>"
  Bus Selector21/21 -> Bauteil_4/21(Lager_Vereinzler_Schritt_Aus)  "<Lager_Vereinzler_Schritt_Aus>"
  Bus Selector21/8 -> Bauteil_4/8(Kran_Zyl_Unten)  "<Kran_Zyl_Unten>"
  Bus Selector21/23 -> Bauteil_4/23(Kran_Zyl_Schritt_Runter)  "<Kran_Zyl_Schritt_Runter>"
  Bus Selector21/6 -> Bauteil_4/6(Kran_Stellung_Stempel)  "<Sensor_Kran_Stellung_Stempel>"
  Bus Selector21/1 -> Bauteil_4/1(Lager_X_Achse)  "<Lager_X_Achse>"
  Bus Selector21/27 -> Bauteil_4/27(Band_Zyl_1_Schritt)  "<Band_Zyl_1_Schritt>"
  Bus Selector21/13 -> Bauteil_4/13(Kran_Drehen_Rechts)  "<Kran_Drehen_Rechts_FS>"
  Bus Selector21/15 -> Bauteil_4/15(Stempel_Halterung_Einfahren)  "<Stempel_Halterung_Einfahren_FS>"
  Bus Selector21/19 -> Bauteil_4/19(Band_Zyl_2_X_Achse)  "<Band_Zyl_2_X_Achse>"
  Bus Selector21/18 -> Bauteil_4/18(Band_Zyl_1_X_Achse)  "<Band_Zyl_1_X_Achse>"
  Bus Selector21/22 -> Bauteil_4/22(Kran_Zyl_Schritt_Hoch)  "<Kran_Zyl_Schritt_Hoch>"
  Bus Selector21/20 -> Bauteil_4/20(Lager_Ver_Ausfahren)  "<Lager_Ver_Ausfahren>"
  Bus Selector21/17 -> Bauteil_4/17(Band_Zurueck)  "<Band_Zurueck_FS>"
  Bus Selector21/24 -> Bauteil_4/24(Kran_Drehen_Schritt)  "<Kran_Drehen_Schritt>"
  Bus Selector21/14 -> Bauteil_4/14(Stempel_Halterung_Ausfahren)  "<Stempel_Halterung_Ausfahren_FS>"
  Bus Selector21/16 -> Bauteil_4/16(Band_Vor)  "<Band_Vor_FS>"
  Bus Selector21/25 -> Bauteil_4/25(Stempel_Halterung_Schritt_Aus)  "<Stempel_Halterung_Schritt_Aus>"
  Bus Selector21/2 -> Bauteil_4/2(Lager_Ver_Eingefahren)  "<Lager_Ver_Eingefahren>"
  Bus Selector21/26 -> Bauteil_4/26(Stempel_Halterung_Schritt_Ein)  "<Stempel_Halterung_Schritt_Ein>"
  Bus Selector21/9 -> Bauteil_4/9(Kran_Sauger)  "<Kran_Sauger>"
  Bus Selector21/29 -> Bauteil_4/29(Band_Geschwindigkeit)  "<Band_Geschwindigkeit>"
  Bus Selector21/12 -> Bauteil_4/12(Kran_Drehen_Links)  "<Kran_Drehen_Links_FS>"
  Bus Selector21/5 -> Bauteil_4/5(Kran_Stellung_Band)  "<Sensor_Kran_Stellung_Band>"
  Bus Selector23/10 -> Bauteil_5/10(Kran_Hochheben)  "<Kran_Hochheben>"
  Bus Selector23/28 -> Bauteil_5/28(Band_Zyl_2_Schritt)  "<Band_Zyl_2_Schritt>"
  Bus Selector23/11 -> Bauteil_5/11(Kran_Runterlassen)  "<Kran_Runterlassen>"
  Bus Selector23/7 -> Bauteil_5/7(Kran_Zyl_Oben)  "<Kran_Zyl_Oben>"
  Bus Selector23/3 -> Bauteil_5/3(Lager_Ver_Ausgefahren)  "<Lager_Ver_Ausgefahren>"
  Bus Selector23/4 -> Bauteil_5/4(Kran_Stellung_Lager)  "<Sensor_Kran_Stellung_Lager>"
  Bus Selector23/30 -> Bauteil_5/30(Bauteil_Fallgeschwindigkeit)  "<Bauteil_Fallgeschwindigkeit>"
  Bus Selector23/21 -> Bauteil_5/21(Lager_Vereinzler_Schritt_Aus)  "<Lager_Vereinzler_Schritt_Aus>"
  Bus Selector23/8 -> Bauteil_5/8(Kran_Zyl_Unten)  "<Kran_Zyl_Unten>"
  Bus Selector23/23 -> Bauteil_5/23(Kran_Zyl_Schritt_Runter)  "<Kran_Zyl_Schritt_Runter>"
  Bus Selector23/6 -> Bauteil_5/6(Kran_Stellung_Stempel)  "<Sensor_Kran_Stellung_Stempel>"
  Bus Selector23/1 -> Bauteil_5/1(Lager_X_Achse)  "<Lager_X_Achse>"
  Bus Selector23/27 -> Bauteil_5/27(Band_Zyl_1_Schritt)  "<Band_Zyl_1_Schritt>"
  Bus Selector23/13 -> Bauteil_5/13(Kran_Drehen_Rechts)  "<Kran_Drehen_Rechts_FS>"
  Bus Selector23/15 -> Bauteil_5/15(Stempel_Halterung_Einfahren)  "<Stempel_Halterung_Einfahren_FS>"
  Bus Selector23/19 -> Bauteil_5/19(Band_Zyl_2_X_Achse)  "<Band_Zyl_2_X_Achse>"
  Bus Selector23/18 -> Bauteil_5/18(Band_Zyl_1_X_Achse)  "<Band_Zyl_1_X_Achse>"
  Bus Selector23/22 -> Bauteil_5/22(Kran_Zyl_Schritt_Hoch)  "<Kran_Zyl_Schritt_Hoch>"
  Bus Selector23/20 -> Bauteil_5/20(Lager_Ver_Ausfahren)  "<Lager_Ver_Ausfahren>"
  Bus Selector23/17 -> Bauteil_5/17(Band_Zurueck)  "<Band_Zurueck_FS>"
  Bus Selector23/24 -> Bauteil_5/24(Kran_Drehen_Schritt)  "<Kran_Drehen_Schritt>"
  Bus Selector23/14 -> Bauteil_5/14(Stempel_Halterung_Ausfahren)  "<Stempel_Halterung_Ausfahren_FS>"
  Bus Selector23/16 -> Bauteil_5/16(Band_Vor)  "<Band_Vor_FS>"
  Bus Selector23/25 -> Bauteil_5/25(Stempel_Halterung_Schritt_Aus)  "<Stempel_Halterung_Schritt_Aus>"
  Bus Selector23/2 -> Bauteil_5/2(Lager_Ver_Eingefahren)  "<Lager_Ver_Eingefahren>"
  Bus Selector23/26 -> Bauteil_5/26(Stempel_Halterung_Schritt_Ein)  "<Stempel_Halterung_Schritt_Ein>"
  Bus Selector23/9 -> Bauteil_5/9(Kran_Sauger)  "<Kran_Sauger>"
  Bus Selector23/29 -> Bauteil_5/29(Band_Geschwindigkeit)  "<Band_Geschwindigkeit>"
  Bus Selector23/12 -> Bauteil_5/12(Kran_Drehen_Links)  "<Kran_Drehen_Links_FS>"
  Bus Selector23/5 -> Bauteil_5/5(Kran_Stellung_Band)  "<Sensor_Kran_Stellung_Band>"
  Bus Selector25/10 -> Bauteil_6/10(Kran_Hochheben)  "<Kran_Hochheben>"
  Bus Selector25/28 -> Bauteil_6/28(Band_Zyl_2_Schritt)  "<Band_Zyl_2_Schritt>"
  Bus Selector25/11 -> Bauteil_6/11(Kran_Runterlassen)  "<Kran_Runterlassen>"
  Bus Selector25/7 -> Bauteil_6/7(Kran_Zyl_Oben)  "<Kran_Zyl_Oben>"
  Bus Selector25/3 -> Bauteil_6/3(Lager_Ver_Ausgefahren)  "<Lager_Ver_Ausgefahren>"
  Bus Selector25/4 -> Bauteil_6/4(Kran_Stellung_Lager)  "<Sensor_Kran_Stellung_Lager>"
  Bus Selector25/30 -> Bauteil_6/30(Bauteil_Fallgeschwindigkeit)  "<Bauteil_Fallgeschwindigkeit>"
  Bus Selector25/21 -> Bauteil_6/21(Lager_Vereinzler_Schritt_Aus)  "<Lager_Vereinzler_Schritt_Aus>"
  Bus Selector25/8 -> Bauteil_6/8(Kran_Zyl_Unten)  "<Kran_Zyl_Unten>"
  Bus Selector25/23 -> Bauteil_6/23(Kran_Zyl_Schritt_Runter)  "<Kran_Zyl_Schritt_Runter>"
  Bus Selector25/6 -> Bauteil_6/6(Kran_Stellung_Stempel)  "<Sensor_Kran_Stellung_Stempel>"
  Bus Selector25/1 -> Bauteil_6/1(Lager_X_Achse)  "<Lager_X_Achse>"
  Bus Selector25/27 -> Bauteil_6/27(Band_Zyl_1_Schritt)  "<Band_Zyl_1_Schritt>"
  Bus Selector25/13 -> Bauteil_6/13(Kran_Drehen_Rechts)  "<Kran_Drehen_Rechts_FS>"
  Bus Selector25/15 -> Bauteil_6/15(Stempel_Halterung_Einfahren)  "<Stempel_Halterung_Einfahren_FS>"
  Bus Selector25/19 -> Bauteil_6/19(Band_Zyl_2_X_Achse)  "<Band_Zyl_2_X_Achse>"
  Bus Selector25/18 -> Bauteil_6/18(Band_Zyl_1_X_Achse)  "<Band_Zyl_1_X_Achse>"
  Bus Selector25/22 -> Bauteil_6/22(Kran_Zyl_Schritt_Hoch)  "<Kran_Zyl_Schritt_Hoch>"
  Bus Selector25/20 -> Bauteil_6/20(Lager_Ver_Ausfahren)  "<Lager_Ver_Ausfahren>"
  Bus Selector25/17 -> Bauteil_6/17(Band_Zurueck)  "<Band_Zurueck_FS>"
  Bus Selector25/24 -> Bauteil_6/24(Kran_Drehen_Schritt)  "<Kran_Drehen_Schritt>"
  Bus Selector25/14 -> Bauteil_6/14(Stempel_Halterung_Ausfahren)  "<Stempel_Halterung_Ausfahren_FS>"
  Bus Selector25/16 -> Bauteil_6/16(Band_Vor)  "<Band_Vor_FS>"
  Bus Selector25/25 -> Bauteil_6/25(Stempel_Halterung_Schritt_Aus)  "<Stempel_Halterung_Schritt_Aus>"
  Bus Selector25/2 -> Bauteil_6/2(Lager_Ver_Eingefahren)  "<Lager_Ver_Eingefahren>"
  Bus Selector25/26 -> Bauteil_6/26(Stempel_Halterung_Schritt_Ein)  "<Stempel_Halterung_Schritt_Ein>"
  Bus Selector25/9 -> Bauteil_6/9(Kran_Sauger)  "<Kran_Sauger>"
  Bus Selector25/29 -> Bauteil_6/29(Band_Geschwindigkeit)  "<Band_Geschwindigkeit>"
  Bus Selector25/12 -> Bauteil_6/12(Kran_Drehen_Links)  "<Kran_Drehen_Links_FS>"
  Bus Selector25/5 -> Bauteil_6/5(Kran_Stellung_Band)  "<Sensor_Kran_Stellung_Band>"
  Bus Selector31/10 -> Bauteil_7/10(Kran_Hochheben)  "<Kran_Hochheben>"
  Bus Selector31/28 -> Bauteil_7/28(Band_Zyl_2_Schritt)  "<Band_Zyl_2_Schritt>"
  Bus Selector31/11 -> Bauteil_7/11(Kran_Runterlassen)  "<Kran_Runterlassen>"
  Bus Selector31/7 -> Bauteil_7/7(Kran_Zyl_Oben)  "<Kran_Zyl_Oben>"
  Bus Selector31/3 -> Bauteil_7/3(Lager_Ver_Ausgefahren)  "<Lager_Ver_Ausgefahren>"
  Bus Selector31/4 -> Bauteil_7/4(Kran_Stellung_Lager)  "<Sensor_Kran_Stellung_Lager>"
  Bus Selector31/30 -> Bauteil_7/30(Bauteil_Fallgeschwindigkeit)  "<Bauteil_Fallgeschwindigkeit>"
  Bus Selector31/21 -> Bauteil_7/21(Lager_Vereinzler_Schritt_Aus)  "<Lager_Vereinzler_Schritt_Aus>"
  Bus Selector31/8 -> Bauteil_7/8(Kran_Zyl_Unten)  "<Kran_Zyl_Unten>"
  Bus Selector31/23 -> Bauteil_7/23(Kran_Zyl_Schritt_Runter)  "<Kran_Zyl_Schritt_Runter>"
  Bus Selector31/6 -> Bauteil_7/6(Kran_Stellung_Stempel)  "<Sensor_Kran_Stellung_Stempel>"
  Bus Selector31/1 -> Bauteil_7/1(Lager_X_Achse)  "<Lager_X_Achse>"
  Bus Selector31/27 -> Bauteil_7/27(Band_Zyl_1_Schritt)  "<Band_Zyl_1_Schritt>"
  Bus Selector31/13 -> Bauteil_7/13(Kran_Drehen_Rechts)  "<Kran_Drehen_Rechts_FS>"
  Bus Selector31/15 -> Bauteil_7/15(Stempel_Halterung_Einfahren)  "<Stempel_Halterung_Einfahren_FS>"
  Bus Selector31/19 -> Bauteil_7/19(Band_Zyl_2_X_Achse)  "<Band_Zyl_2_X_Achse>"
  Bus Selector31/18 -> Bauteil_7/18(Band_Zyl_1_X_Achse)  "<Band_Zyl_1_X_Achse>"
  Bus Selector31/22 -> Bauteil_7/22(Kran_Zyl_Schritt_Hoch)  "<Kran_Zyl_Schritt_Hoch>"
  Bus Selector31/20 -> Bauteil_7/20(Lager_Ver_Ausfahren)  "<Lager_Ver_Ausfahren>"
  Bus Selector31/17 -> Bauteil_7/17(Band_Zurueck)  "<Band_Zurueck_FS>"
  Bus Selector31/24 -> Bauteil_7/24(Kran_Drehen_Schritt)  "<Kran_Drehen_Schritt>"
  Bus Selector31/14 -> Bauteil_7/14(Stempel_Halterung_Ausfahren)  "<Stempel_Halterung_Ausfahren_FS>"
  Bus Selector31/16 -> Bauteil_7/16(Band_Vor)  "<Band_Vor_FS>"
  Bus Selector31/25 -> Bauteil_7/25(Stempel_Halterung_Schritt_Aus)  "<Stempel_Halterung_Schritt_Aus>"
  Bus Selector31/2 -> Bauteil_7/2(Lager_Ver_Eingefahren)  "<Lager_Ver_Eingefahren>"
  Bus Selector31/26 -> Bauteil_7/26(Stempel_Halterung_Schritt_Ein)  "<Stempel_Halterung_Schritt_Ein>"
  Bus Selector31/9 -> Bauteil_7/9(Kran_Sauger)  "<Kran_Sauger>"
  Bus Selector31/29 -> Bauteil_7/29(Band_Geschwindigkeit)  "<Band_Geschwindigkeit>"
  Bus Selector31/12 -> Bauteil_7/12(Kran_Drehen_Links)  "<Kran_Drehen_Links_FS>"
  Bus Selector31/5 -> Bauteil_7/5(Kran_Stellung_Band)  "<Sensor_Kran_Stellung_Band>"
  Bus Selector32/10 -> Bauteil_8/10(Kran_Hochheben)  "<Kran_Hochheben>"
  Bus Selector32/28 -> Bauteil_8/28(Band_Zyl_2_Schritt)  "<Band_Zyl_2_Schritt>"
  Bus Selector32/11 -> Bauteil_8/11(Kran_Runterlassen)  "<Kran_Runterlassen>"
  Bus Selector32/7 -> Bauteil_8/7(Kran_Zyl_Oben)  "<Kran_Zyl_Oben>"
  Bus Selector32/3 -> Bauteil_8/3(Lager_Ver_Ausgefahren)  "<Lager_Ver_Ausgefahren>"
  Bus Selector32/4 -> Bauteil_8/4(Kran_Stellung_Lager)  "<Sensor_Kran_Stellung_Lager>"
  Bus Selector32/30 -> Bauteil_8/30(Bauteil_Fallgeschwindigkeit)  "<Bauteil_Fallgeschwindigkeit>"
  Bus Selector32/21 -> Bauteil_8/21(Lager_Vereinzler_Schritt_Aus)  "<Lager_Vereinzler_Schritt_Aus>"
  Bus Selector32/8 -> Bauteil_8/8(Kran_Zyl_Unten)  "<Kran_Zyl_Unten>"
  Bus Selector32/23 -> Bauteil_8/23(Kran_Zyl_Schritt_Runter)  "<Kran_Zyl_Schritt_Runter>"
  Bus Selector32/6 -> Bauteil_8/6(Kran_Stellung_Stempel)  "<Sensor_Kran_Stellung_Stempel>"
  Bus Selector32/1 -> Bauteil_8/1(Lager_X_Achse)  "<Lager_X_Achse>"
  Bus Selector32/27 -> Bauteil_8/27(Band_Zyl_1_Schritt)  "<Band_Zyl_1_Schritt>"
  Bus Selector32/13 -> Bauteil_8/13(Kran_Drehen_Rechts)  "<Kran_Drehen_Rechts_FS>"
  Bus Selector32/15 -> Bauteil_8/15(Stempel_Halterung_Einfahren)  "<Stempel_Halterung_Einfahren_FS>"
  Bus Selector32/19 -> Bauteil_8/19(Band_Zyl_2_X_Achse)  "<Band_Zyl_2_X_Achse>"
  Bus Selector32/18 -> Bauteil_8/18(Band_Zyl_1_X_Achse)  "<Band_Zyl_1_X_Achse>"
  Bus Selector32/22 -> Bauteil_8/22(Kran_Zyl_Schritt_Hoch)  "<Kran_Zyl_Schritt_Hoch>"
  Bus Selector32/20 -> Bauteil_8/20(Lager_Ver_Ausfahren)  "<Lager_Ver_Ausfahren>"
  Bus Selector32/17 -> Bauteil_8/17(Band_Zurueck)  "<Band_Zurueck_FS>"
  Bus Selector32/24 -> Bauteil_8/24(Kran_Drehen_Schritt)  "<Kran_Drehen_Schritt>"
  Bus Selector32/14 -> Bauteil_8/14(Stempel_Halterung_Ausfahren)  "<Stempel_Halterung_Ausfahren_FS>"
  Bus Selector32/16 -> Bauteil_8/16(Band_Vor)  "<Band_Vor_FS>"
  Bus Selector32/25 -> Bauteil_8/25(Stempel_Halterung_Schritt_Aus)  "<Stempel_Halterung_Schritt_Aus>"
  Bus Selector32/2 -> Bauteil_8/2(Lager_Ver_Eingefahren)  "<Lager_Ver_Eingefahren>"
  Bus Selector32/26 -> Bauteil_8/26(Stempel_Halterung_Schritt_Ein)  "<Stempel_Halterung_Schritt_Ein>"
  Bus Selector32/9 -> Bauteil_8/9(Kran_Sauger)  "<Kran_Sauger>"
  Bus Selector32/29 -> Bauteil_8/29(Band_Geschwindigkeit)  "<Band_Geschwindigkeit>"
  Bus Selector32/12 -> Bauteil_8/12(Kran_Drehen_Links)  "<Kran_Drehen_Links_FS>"
  Bus Selector32/5 -> Bauteil_8/5(Kran_Stellung_Band)  "<Sensor_Kran_Stellung_Band>"
  Bus Selector34/10 -> Bauteil_9/10(Kran_Hochheben)  "<Kran_Hochheben>"
  Bus Selector34/28 -> Bauteil_9/28(Band_Zyl_2_Schritt)  "<Band_Zyl_2_Schritt>"
  Bus Selector34/11 -> Bauteil_9/11(Kran_Runterlassen)  "<Kran_Runterlassen>"
  Bus Selector34/7 -> Bauteil_9/7(Kran_Zyl_Oben)  "<Kran_Zyl_Oben>"
  Bus Selector34/3 -> Bauteil_9/3(Lager_Ver_Ausgefahren)  "<Lager_Ver_Ausgefahren>"
  Bus Selector34/4 -> Bauteil_9/4(Kran_Stellung_Lager)  "<Sensor_Kran_Stellung_Lager>"
  Bus Selector34/30 -> Bauteil_9/30(Bauteil_Fallgeschwindigkeit)  "<Bauteil_Fallgeschwindigkeit>"
  Bus Selector34/21 -> Bauteil_9/21(Lager_Vereinzler_Schritt_Aus)  "<Lager_Vereinzler_Schritt_Aus>"
  Bus Selector34/8 -> Bauteil_9/8(Kran_Zyl_Unten)  "<Kran_Zyl_Unten>"
  Bus Selector34/23 -> Bauteil_9/23(Kran_Zyl_Schritt_Runter)  "<Kran_Zyl_Schritt_Runter>"
  Bus Selector34/6 -> Bauteil_9/6(Kran_Stellung_Stempel)  "<Sensor_Kran_Stellung_Stempel>"
  Bus Selector34/1 -> Bauteil_9/1(Lager_X_Achse)  "<Lager_X_Achse>"
  Bus Selector34/27 -> Bauteil_9/27(Band_Zyl_1_Schritt)  "<Band_Zyl_1_Schritt>"
  Bus Selector34/13 -> Bauteil_9/13(Kran_Drehen_Rechts)  "<Kran_Drehen_Rechts_FS>"
  Bus Selector34/15 -> Bauteil_9/15(Stempel_Halterung_Einfahren)  "<Stempel_Halterung_Einfahren_FS>"
  Bus Selector34/19 -> Bauteil_9/19(Band_Zyl_2_X_Achse)  "<Band_Zyl_2_X_Achse>"
  Bus Selector34/18 -> Bauteil_9/18(Band_Zyl_1_X_Achse)  "<Band_Zyl_1_X_Achse>"
  Bus Selector34/22 -> Bauteil_9/22(Kran_Zyl_Schritt_Hoch)  "<Kran_Zyl_Schritt_Hoch>"
  Bus Selector34/20 -> Bauteil_9/20(Lager_Ver_Ausfahren)  "<Lager_Ver_Ausfahren>"
  Bus Selector34/17 -> Bauteil_9/17(Band_Zurueck)  "<Band_Zurueck_FS>"
  Bus Selector34/24 -> Bauteil_9/24(Kran_Drehen_Schritt)  "<Kran_Drehen_Schritt>"
  Bus Selector34/14 -> Bauteil_9/14(Stempel_Halterung_Ausfahren)  "<Stempel_Halterung_Ausfahren_FS>"
  Bus Selector34/16 -> Bauteil_9/16(Band_Vor)  "<Band_Vor_FS>"
  Bus Selector34/25 -> Bauteil_9/25(Stempel_Halterung_Schritt_Aus)  "<Stempel_Halterung_Schritt_Aus>"
  Bus Selector34/2 -> Bauteil_9/2(Lager_Ver_Eingefahren)  "<Lager_Ver_Eingefahren>"
  Bus Selector34/26 -> Bauteil_9/26(Stempel_Halterung_Schritt_Ein)  "<Stempel_Halterung_Schritt_Ein>"
  Bus Selector34/9 -> Bauteil_9/9(Kran_Sauger)  "<Kran_Sauger>"
  Bus Selector34/29 -> Bauteil_9/29(Band_Geschwindigkeit)  "<Band_Geschwindigkeit>"
  Bus Selector34/12 -> Bauteil_9/12(Kran_Drehen_Links)  "<Kran_Drehen_Links_FS>"
  Bus Selector34/5 -> Bauteil_9/5(Kran_Stellung_Band)  "<Sensor_Kran_Stellung_Band>"
  Bus Creator2/1 -> Bus Creator10/1, Bus Selector8/1, Bus Selector27/1, Bus Selector9/1, Bus Selector28/1, Bus Selector21/1, Bus Selector23/1, Bus Selector30/1, Bus Selector25/1, Bus Selector31/1, Bus Selector37/1, Bus Selector38/1, Bus Selector34/1, Bus Selector32/1, Bus Selector36/1, Bus Selector29/1, Bus Selector2/1, Bus Selector1/1, Bus Selector6/1  "Stempelanlage"
  Bus Creator18/1 -> Stempel_Schalter/1  "Stempel_Schalter"
  Bus Creator19/1 -> Lager_Schalter/1  "Lager_Schalter"
  Bus Creator36/1 -> Band_Schalter/1  "Band_Schalter"
  Lager_Source/1 -> Rate Transition1/1
  Lager_Source/2 -> Rate Transition2/1  "Lager_NotAus"
  Stempel_Source/1 -> Rate Transition3/1
  Stempel_Source/2 -> Rate Transition4/1
  Band_Source/1 -> Rate Transition5/1  "Band_Start"
  Band_Source/2 -> Rate Transition6/1
  Rate Transition2/1 -> Bus Creator19/2, Logical Operator/2  "Lager_Notaus"
  Logical Operator/1 -> Bus Creator2/2  "Notaus_Switch"
  Subsystem/1(BT_Y_Out) -> Bus Creator8/1  "BT_1_Y_Achse"
  Bus Selector6/1 -> Subsystem/1(Notaus_Knopf)  "<Notaus_Switch>"
  Subsystem8/1(BT_Y_Out) -> Bus Creator12/1  "BT_2_Y_Achse"
  Subsystem1/1(BT_Y_Out) -> Bus Creator22/1  "BT_3_Y_Achse"
  Subsystem2/1(BT_Y_Out) -> Bus Creator25/1  "BT_4_Y_Achse"
  Subsystem3/1(BT_Y_Out) -> Bus Creator27/1  "BT_5_Y_Achse"
  Subsystem4/1(BT_Y_Out) -> Bus Creator28/1  "BT_6_Y_Achse"
  Subsystem5/1(BT_Y_Out) -> Bus Creator30/1  "BT_7_Y_Achse"
  Subsystem6/1(BT_Y_Out) -> Bus Creator32/1  "BT_8_Y_Achse"
  Subsystem7/1(BT_Y_Out) -> Bus Creator34/1  "BT_9_Y_Achse"
  Bus Selector8/1 -> Subsystem8/1(Notaus_Knopf)  "<Notaus_Switch>"
  Bus Selector27/1 -> Subsystem1/1(Notaus_Knopf)  "<Notaus_Switch>"
  Bus Selector28/1 -> Subsystem2/1(Notaus_Knopf)  "<Notaus_Switch>"
  Bus Selector29/1 -> Subsystem3/1(Notaus_Knopf)  "<Notaus_Switch>"
  Bus Selector30/1 -> Subsystem4/1(Notaus_Knopf)  "<Notaus_Switch>"
  Bus Selector36/1 -> Subsystem5/1(Notaus_Knopf)  "<Notaus_Switch>"
  Bus Selector37/1 -> Subsystem6/1(Notaus_Knopf)  "<Notaus_Switch>"
  Bus Selector38/1 -> Subsystem7/1(Notaus_Knopf)  "<Notaus_Switch>"
  Subsystem/3(BT_Lager_Out) -> Bus Creator8/3  "BT_1_Lager"
  Subsystem/2(BT_Angesaugt_Out) -> Bus Creator8/2  "Kran_Sauger_BT_1"
  Subsystem8/2(BT_Angesaugt_Out) -> Bus Creator12/2  "Kran_Sauger_BT_2"
  Subsystem8/3(BT_Lager_Out) -> Bus Creator12/3  "BT_2_Lager"
  Subsystem1/2(BT_Angesaugt_Out) -> Bus Creator22/2  "Kran_Sauger_BT_3"
  Subsystem1/3(BT_Lager_Out) -> Bus Creator22/3  "BT_3_Lager"
  Subsystem2/3(BT_Lager_Out) -> Bus Creator25/3  "BT_4_Lager"
  Subsystem2/2(BT_Angesaugt_Out) -> Bus Creator25/2  "Kran_Sauger_BT_4"
  Subsystem3/3(BT_Lager_Out) -> Bus Creator27/3  "BT_5_Lager"
  Subsystem3/2(BT_Angesaugt_Out) -> Bus Creator27/2  "Kran_Sauger_BT_5"
  Subsystem4/2(BT_Angesaugt_Out) -> Bus Creator28/2  "Kran_Sauger_BT_6"
  Subsystem4/3(BT_Lager_Out) -> Bus Creator28/3  "BT_6_Lager"
  Subsystem5/3(BT_Lager_Out) -> Bus Creator30/3  "BT_7_Lager"
  Subsystem5/2(BT_Angesaugt_Out) -> Bus Creator30/2  "Kran_Sauger_BT_7"
  Subsystem6/2(BT_Angesaugt_Out) -> Bus Creator32/2  "Kran_Sauger_BT_8"
  Subsystem6/3(BT_Lager_Out) -> Bus Creator32/3  "BT_8_Lager"
  Subsystem7/2(BT_Angesaugt_Out) -> Bus Creator34/2  "Kran_Sauger_BT_9"
  Subsystem7/3(BT_Lager_Out) -> Bus Creator34/3  "BT_9_Lager"
  Subsystem/4(BT_Bereit_Out) -> Bus Creator8/4  "BT_1_Bereit"
  Subsystem8/4(BT_Bereit_Out) -> Bus Creator12/4  "BT_2_Bereit"
  Subsystem1/4(BT_Bereit_Out) -> Bus Creator22/4  "BT_3_Bereit"
  Subsystem2/4(BT_Bereit_Out) -> Bus Creator25/4  "BT_4_Bereit"
  Subsystem3/4(BT_Bereit_Out) -> Bus Creator27/4  "BT_5_Bereit"
  Subsystem4/4(BT_Bereit_Out) -> Bus Creator28/4  "BT_6_Bereit"
  Subsystem5/4(BT_Bereit_Out) -> Bus Creator30/4  "BT_7_Bereit"
  Subsystem6/4(BT_Bereit_Out) -> Bus Creator32/4  "BT_8_Bereit"
  Subsystem7/4(BT_Bereit_Out) -> Bus Creator34/4  "BT_9_Bereit"
